simulink model "PID_sintonization"  (R2024a)
settings: Solver=VariableStepAuto  StartTime=0.0  StopTime=500.0  RelTol=1e-3
values from neighbouring files (symbols this model uses):
  q1 = entr(3)    [directKinematics.m]
  q2 = entr(4)    [directKinematics.m]
undefined symbols (not defined in the file or in its folder): telescopeParam
libraries: simulink_extras x4
settings Model: Creator=b_ant  LastModifiedBy=b_ant

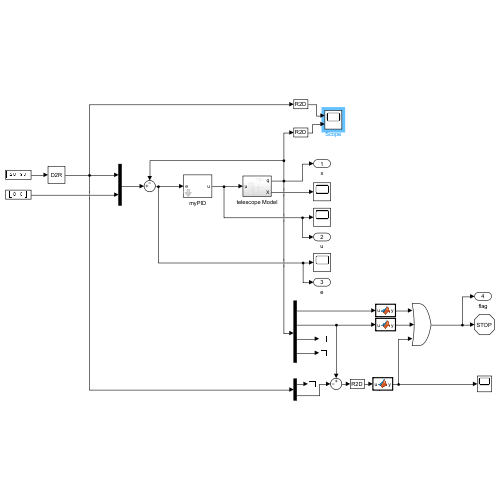
[thumbnail: Simulink's stored preview of the top-level diagram]
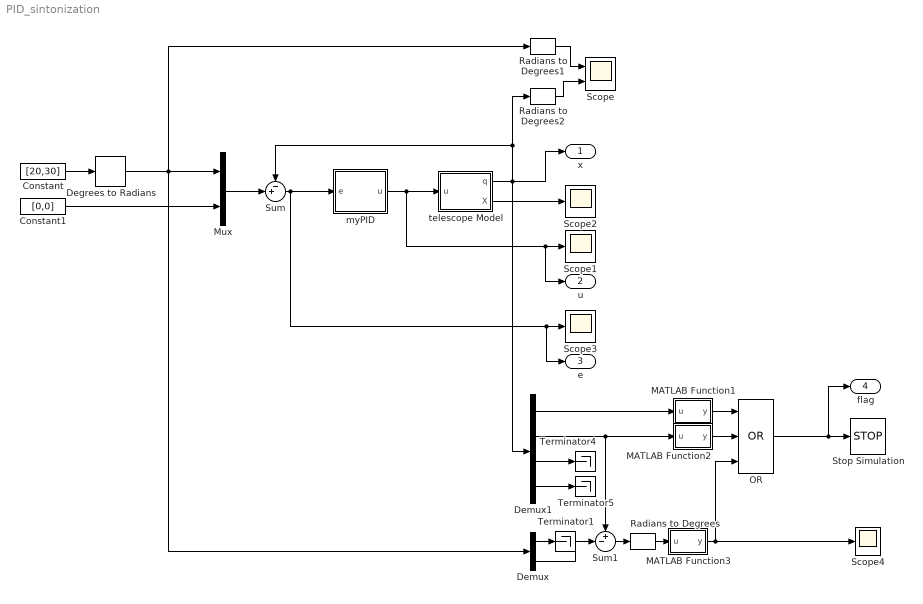
== system PID_sintonization ==
  Constant : Constant  Value=[20,30]
  Constant1 : Constant  Value=[0,0]
  Degrees to Radians : simulink_extras/Transformations/Degrees to Radians
  Demux : Demux  Outputs=2
  Demux1 : Demux
  MATLAB Function1 : MATLAB Function  TreatAsAtomicUnit=on
  MATLAB Function2 : MATLAB Function  TreatAsAtomicUnit=on
  MATLAB Function3 : MATLAB Function  TreatAsAtomicUnit=on
  Mux : Mux  Inputs=2
  OR : Logic  Operator=OR  Inputs=3  IconShape=distinctive  AllPortsSameDT=off  OutDataTypeStr=boolean
  Radians to Degrees : simulink_extras/Transformations/Radians to Degrees
  Radians to Degrees1 : simulink_extras/Transformations/Radians to Degrees
  Radians to Degrees2 : simulink_extras/Transformations/Radians to Degrees
  Scope : Scope  NumInputPorts=2
  Scope{1..4} (4 alike) : Scope
  Stop Simulation : Stop
  Sum : Sum  Inputs=-+|
  Sum1 : Sum  Inputs=+-|
  Terminator1 : Terminator
  Terminator4 : Terminator
  Terminator5 : Terminator
  myPID : Subsystem
  telescope Model : Subsystem
  x : Outport
  u : Outport  Port=2
  e : Outport  Port=3
  flag : Outport  Port=4
  wires:
  Demux1/2 -> Sum1/1, MATLAB Function2/1(u)
  MATLAB Function1/1(y) -> OR/1
  myPID/1(u) -> u/1, Scope1/1, telescope Model/1(u)
  Constant/1 -> Degrees to Radians/1
  telescope Model/2(X) -> Scope2/1
  Constant1/1 -> Mux/2
  Demux1/3 -> Terminator4/1
  Demux1/1 -> MATLAB Function1/1(u)
  Mux/1 -> Sum/2
  Sum/1 -> myPID/1(e), e/1, Scope3/1
  telescope Model/1(q) -> Radians to Degrees2/1, Sum/1, x/1, Demux1/1
  Demux1/4 -> Terminator5/1
  MATLAB Function2/1(y) -> OR/2
  OR/1 -> flag/1, Stop Simulation/1
  Degrees to Radians/1 -> Demux/1, Radians to Degrees1/1, Mux/1
  MATLAB Function3/1(y) -> Scope4/1, OR/3
  Sum1/1 -> Radians to Degrees/1
  Demux/2 -> Sum1/2
  Radians to Degrees/1 -> MATLAB Function3/1(u)
  Demux/1 -> Terminator1/1
  Radians to Degrees1/1 -> Scope/1
  Radians to Degrees2/1 -> Scope/2

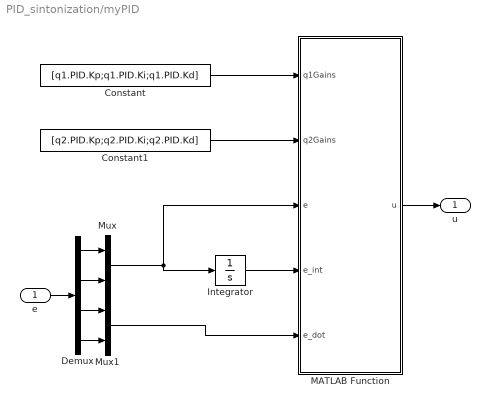
== system PID_sintonization/myPID ==
  e : Inport
  Constant : Constant  Value=[q1.PID.Kp;q1.PID.Ki;q1.PID.Kd]
  Constant1 : Constant  Value=[q2.PID.Kp;q2.PID.Ki;q2.PID.Kd]
  Demux : Demux
  Integrator : Integrator
  MATLAB Function : MATLAB Function  TreatAsAtomicUnit=on
  Mux : Mux  Inputs=2
  Mux1 : Mux  Inputs=2
  u : Outport
  wires:
  MATLAB Function/1(u) -> u/1
  e/1 -> Demux/1
  Mux/1 -> Integrator/1, MATLAB Function/3(e)
  Integrator/1 -> MATLAB Function/4(e_int)
  Constant/1 -> MATLAB Function/1(q1Gains)
  Demux/1 -> Mux/1
  Demux/2 -> Mux/2
  Demux/3 -> Mux1/1
  Demux/4 -> Mux1/2
  Mux1/1 -> MATLAB Function/5(e_dot)
  Constant1/1 -> MATLAB Function/2(q2Gains)

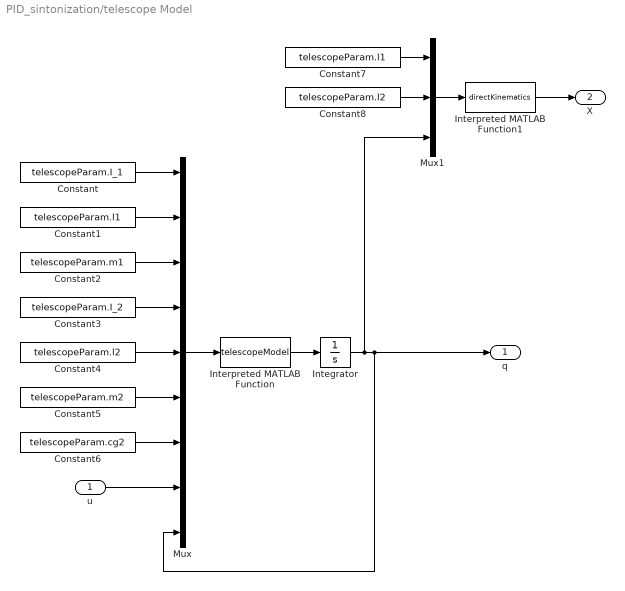
== system PID_sintonization/telescope Model ==
  u : Inport
  Constant : Constant  Value=telescopeParam.I_1
  Constant1 : Constant  Value=telescopeParam.l1
  Constant2 : Constant  Value=telescopeParam.m1
  Constant3 : Constant  Value=telescopeParam.I_2
  Constant4 : Constant  Value=telescopeParam.l2
  Constant5 : Constant  Value=telescopeParam.m2
  Constant6 : Constant  Value=telescopeParam.cg2
  Constant7 : Constant  Value=telescopeParam.l1
  Constant8 : Constant  Value=telescopeParam.l2
  Integrator : Integrator  InitialCondition=[0,0,0,0]'
  Interpreted MATLAB Function : MATLABFcn  MATLABFcn=telescopeModel
  Interpreted MATLAB Function1 : MATLABFcn  MATLABFcn=directKinematics
  Mux : Mux  Inputs=9
  Mux1 : Mux  Inputs=3
  q : Outport
  X : Outport  Port=2
  wires:
  Mux/1 -> Interpreted MATLAB Function/1
  Constant4/1 -> Mux/5
  Constant3/1 -> Mux/4
  u/1 -> Mux/8
  Constant/1 -> Mux/1
  Constant5/1 -> Mux/6
  Constant1/1 -> Mux/2
  Constant2/1 -> Mux/3
  Integrator/1 -> q/1, Mux/9, Mux1/3
  Interpreted MATLAB Function/1 -> Integrator/1
  Constant6/1 -> Mux/7
  Mux1/1 -> Interpreted MATLAB Function1/1
  Constant7/1 -> Mux1/1
  Constant8/1 -> Mux1/2
  Interpreted MATLAB Function1/1 -> X/1

== matlab function PID_sintonization/MATLAB Function1 ==
  data: u input; y output
function y = fcn(u)
if abs(u)>4
 y = 1;
else
    y=0;
end
end

== matlab function PID_sintonization/MATLAB Function3 ==
  data: u input; y output
function y = fcn(u)
    if (u) >  2.437
        y = 1;
    else
        y = 0;
    end
end

== matlab function PID_sintonization/MATLAB Function2 ==
  data: u input; y output
function y = fcn(u)
if u>4
 y = 1;
else
    y=0;
end
end

== matlab function PID_sintonization/myPID/MATLAB Function ==
  data: q1Gains input; u output; q2Gains input; e input; e_int input; e_dot input
function u  = pid_controller(q1Gains, q2Gains, e, e_int, e_dot) 
    
    kp = diag([q1Gains(1),q2Gains(1)]);
    ki = diag([q1Gains(2),q2Gains(2)]);
    kd = diag([q1Gains(3),q2Gains(3)]);

    %u_p=kp*e+ki*e_int+kd*e_dot;
    u=kp*e+ki*e_int+kd*e_dot;

    %u=[u_p(1);0];
end
